simulink model "power_pmmotor"  (R2013a)
settings: Solver=ode23tb  SolverMode=SingleTasking  StartTime=0.0  StopTime=0.06  RelTol=1e-4
libraries: powerlib x5
Description:
  | Copyright 2008-2013 The MathWorks, Inc.
settings Model: ExtModeTrigMode=oneshot  ExtModeArmWhenConnect=off  ExtModeAutoUpdateStatusClock=off  Creator=MathWorks  LastModifiedBy=batserve
settings DataIOCC: ExternalInput=[]  LimitDataPoints=off  SignalLoggingSaveFormat=ModelDataLogs  SaveOutput=off  SaveTime=off  SignalLoggingName=sigsOut
settings OptimizationCC: BlockReduction=off  BooleanDataType=off  ExpressionDepthLimit=2147483647  InitFltsAndDblsToZero=on  EfficientMapNaN2IntZero=off
settings DebuggingCC: CheckExecutionContextPreStartOutputMsg=on  CheckExecutionContextRuntimeOutputMsg=on  SignalResolutionControl=TryResolveAllWithWarning  SolverPrmCheckMsg=none  MultiTaskDSMMsg=warning  MultiTaskCondExecSysMsg=none  SigSpecEnsureSampleTimeMsg=none  FcnCallInpInsideContextMsg=UseLocalSettings
settings HardwareCC: TargetUnknown=on
settings RTWCC: IncludeERTFirstTime=on
settings GRTTargetCC: CombineOutputUpdateFcns=off  GRTInterface=on

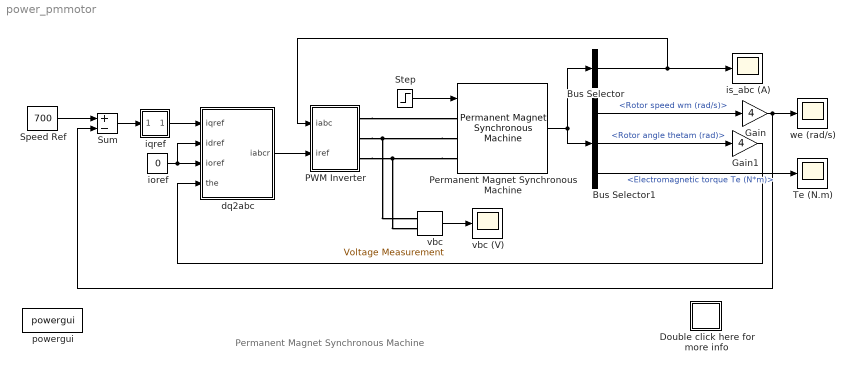
== system power_pmmotor ==
  note: Permanent Magnet Synchronous Machine
  Bus Selector : BusSelector  OutputSignals=Stator current is_a (A),Stator current is_b (A),Stator current is_c (A)  OutputAsBus=on
  Bus Selector1 : BusSelector  OutputSignals=Rotor speed wm (rad/s),Rotor angle thetam (rad),Electromagnetic torque Te (N*m)
  Double click here for more info : Subsystem
      settings: OpenFcn=showdemo(bdroot(gcb))
      mask Display: disp('?')
  Gain : Gain  Gain=4  SaturateOnIntegerOverflow=on  OutDataTypeStr=Inherit: Same as input  ParamDataTypeStr=Inherit: Same as input
  Gain1 : Gain  Gain=4  SaturateOnIntegerOverflow=on  OutDataTypeStr=Inherit: Same as input  ParamDataTypeStr=Inherit: Same as input
  PWM Inverter : Subsystem
  Permanent Magnet Synchronous Machine : powerlib/Machines/Permanent Magnet Synchronous Machine  NbPhases=3  FluxDistribution=Sinusoidal  RotorType=Round  MechanicalLoad=Torque Tm  PresetModel=No  ShowDetailedParameters=on  Resistance=2.875  Inductance=8.5e-3  dqInductances=[8.5e-3,8.5e-3]  La=0.00153  MachineConstant=Flux linkage established by magnets (V.s)  Flux=0.175  VoltageCst=126.966  TorqueCst=1.05  Flat=120  Mechanical=[ 0.8e-3, 0 4]  PolePairs=4  InitialConditions=[0,0, 0,0]  InitialConditions5ph=[0 0 0 0 0 0]  TsPowergui=0  TsBlock=-1  RefAngle=90 degrees behind phase A axis (modified Park)
  Speed Ref : Constant  Value=700
  Step : Step  Time=0.04  Before=3  SampleTime=0
  Sum : Sum  Inputs=+-  SaturateOnIntegerOverflow=on  InputSameDT=on  OutDataTypeStr=Inherit: Same as first input
  Te (N.m) : Scope
      settings: TimeRange=0.06  YMin=-20  YMax=35  DataFormat=Structure
  dq2abc : Subsystem
  ioref : Constant  Value=0
  iqref : Subsystem  mask(PI Controller){I=3, P=40, sat=[-30, 30]}
      mask prompts: I "Integral"; P "Proportional:"; sat "Minimum and maximum outputs:"
      mask init:
      | min=sat(1);max=sat(2);
      mask Display: disp('PI')
  is_abc (A) : Scope
      settings: TimeRange=0.06  YMin=-30  YMax=35  DataFormat=Structure
  powergui : powerlib/powergui  SimulationMode=Continuous  SolverType=Tustin  SampleTime=0  frequency=60  SPID=off  DisableSnubberDevices=off  DisableRonSwitches=off  DisableVfSwitches=off  SwTol=0  Interpol=off  DisplayEquations=off  frequencyindice=0  Pbase=100e6  ErrMax=1e-4  Iterations=50  UnitsV=kV  UnitsW=MW  FunctionMessages=off  echomessages=off  HookPort=off  EnableUseOfTLC=off  x0status=blocks  RestoreLinks=warning  ResistiveCurrentMeasurement=off  Frange=[0:2:500]  Ylog=off  Xlog=on  ShowGrid=off  save=off  variable=ZData  ZoomFFT=on  StartTime=0.0  cycles=1  DisplayStyle=1  fundamental=60  FreqAxis=off  MaxFrequency=1000  frequencyindicesteady=1  RmsSteady=1  display=off  Ts=0  methode=off
  vbc : powerlib/Measurements/Voltage Measurement  Tag=PoWeRsYsTeMmEaSuReMeNt  PhasorSimulation=off  OutputType=Magnitude  PSBequivalent=0
  vbc (V) : Scope
      settings: TimeRange=0.06  YMin=-500  YMax=500  DataFormat=Structure
  we (rad/s) : Scope
      settings: TimeRange=0.06  YMin=0  YMax=800  DataFormat=Structure
  wires:
  ioref/1 -> dq2abc/2(idref), dq2abc/3(ioref)
  Sum/1 -> iqref/1(In_1)
  Speed Ref/1 -> Sum/1
  iqref/1(Out_1) -> dq2abc/1(iqref)
  dq2abc/1(iabcr) -> PWM Inverter/2(iref)
  Bus Selector1/3 -> Te (N.m)/1  "<Electromagnetic torque Te (N*m)>"
  Gain/1 -> we (rad/s)/1, Sum/2
  Gain1/1 -> dq2abc/4(the)
  Step/1 -> Permanent Magnet Synchronous Machine/1
  Permanent Magnet Synchronous Machine/1 -> Bus Selector/1, Bus Selector1/1
  vbc/1 -> vbc (V)/1
  Bus Selector/1 -> PWM Inverter/1(iabc), is_abc (A)/1
  Bus Selector1/1 -> Gain/1  "<Rotor speed wm (rad/s)>"
  Bus Selector1/2 -> Gain1/1  "<Rotor angle thetam (rad)>"
  connections:
  PWM Inverter/RConn1 -- Permanent Magnet Synchronous Machine/LConn1
  Permanent Magnet Synchronous Machine/LConn2 -- PWM Inverter/RConn2 -- vbc/LConn1
  Permanent Magnet Synchronous Machine/LConn3 -- PWM Inverter/RConn3 -- vbc/LConn2

== system power_pmmotor/Double click here for more info ==

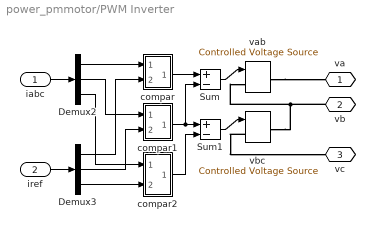
== system power_pmmotor/PWM Inverter ==
  iabc : Inport
  iref : Inport  Port=2
  Demux2 : Demux  Outputs=3
  Demux3 : Demux  Outputs=3
  Sum : Sum  Inputs=+-  SaturateOnIntegerOverflow=on  InputSameDT=on  OutDataTypeStr=Inherit: Same as first input
  Sum1 : Sum  Inputs=+-  SaturateOnIntegerOverflow=on  InputSameDT=on  OutDataTypeStr=Inherit: Same as first input
  compar : Subsystem
  compar1 : Subsystem
  compar2 : Subsystem
  vab : powerlib/Electrical Sources/Controlled Voltage Source  Description=source block  Initialize=on  Source_Type=AC  Amplitude=0  Phase=0  Frequency=0  Measurements=None
      settings: AttributesFormatString=\n
  vbc : powerlib/Electrical Sources/Controlled Voltage Source  Description=source block  Initialize=on  Source_Type=AC  Amplitude=0  Phase=0  Frequency=0  Measurements=None
      settings: AttributesFormatString=\n
  va : PMIOPort  Port=1  Side=Right
  vb : PMIOPort  Port=2  Side=Right
  vc : PMIOPort  Port=3  Side=Right
  wires:
  Demux2/1 -> compar/1(ia)
  Demux2/2 -> compar1/1(ib)
  Demux2/3 -> compar2/1(ic)
  Demux3/3 -> compar2/2(icr)
  Demux3/2 -> compar1/2(ibr)
  Demux3/1 -> compar/2(iar)
  compar/1(va) -> Sum/1
  compar1/1(vb) -> Sum/2, Sum1/1
  compar2/1(vc) -> Sum1/2
  iabc/1 -> Demux2/1
  iref/1 -> Demux3/1
  Sum/1 -> vab/1
  Sum1/1 -> vbc/1
  connections:
  vab/RConn1 -- va/RConn1
  vb/RConn1 -- vab/LConn1 -- vbc/RConn1
  vbc/LConn1 -- vc/RConn1

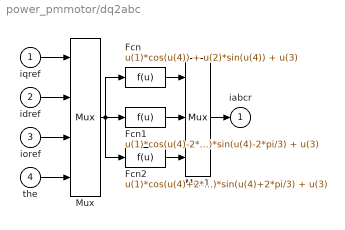
== system power_pmmotor/dq2abc ==
  iqref : Inport
  idref : Inport  Port=2
  ioref : Inport  Port=3
  the : Inport  Port=4
  Fcn : Fcn  Expr=u(1)*cos(u(4)) + u(2)*sin(u(4)) + u(3)
  Fcn1 : Fcn  Expr=u(1)*cos(u(4)-2*pi/3) + u(2)*sin(u(4)-2*pi/3) + u(3)
  Fcn2 : Fcn  Expr=u(1)*cos(u(4)+2*pi/3) + u(2)*sin(u(4)+2*pi/3) + u(3)
  Mux : Mux
  Mux1 : Mux  Inputs=3
  iabcr : Outport  InitialOutput=0
  wires:
  the/1 -> Mux/4
  ioref/1 -> Mux/3
  idref/1 -> Mux/2
  iqref/1 -> Mux/1
  Mux/1 -> Fcn1/1, Fcn2/1, Fcn/1
  Fcn1/1 -> Mux1/2
  Fcn/1 -> Mux1/1
  Fcn2/1 -> Mux1/3
  Mux1/1 -> iabcr/1

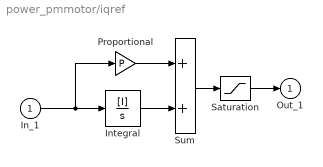
== system power_pmmotor/iqref ==
  In_1 : Inport
  Integral : TransferFcn  Numerator=[I]  Denominator=[1 0]
  Proportional : Gain  Gain=P  SaturateOnIntegerOverflow=on  OutDataTypeStr=Inherit: Same as input  ParamDataTypeStr=Inherit: Same as input
  Saturation : Saturate  UpperLimit=max  LowerLimit=min
  Sum : Sum  SaturateOnIntegerOverflow=on  InputSameDT=on  OutDataTypeStr=Inherit: Same as first input
  Out_1 : Outport  InitialOutput=0
  wires:
  Integral/1 -> Sum/2
  In_1/1 -> Integral/1, Proportional/1
  Proportional/1 -> Sum/1
  Sum/1 -> Saturation/1
  Saturation/1 -> Out_1/1

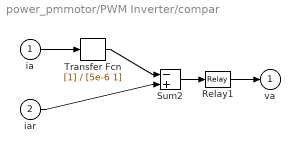
== system power_pmmotor/PWM Inverter/compar ==
  ia : Inport
  iar : Inport  Port=2
  Relay1 : Relay  OnSwitchValue=0.05  OffSwitchValue=-0.05  OnOutputValue=155  OffOutputValue=-155
  Sum2 : Sum  Inputs=-+  SaturateOnIntegerOverflow=on  InputSameDT=on  OutDataTypeStr=Inherit: Same as first input
  Transfer Fcn : TransferFcn  Denominator=[5e-6 1]
  va : Outport  InitialOutput=0
  wires:
  iar/1 -> Sum2/2
  Sum2/1 -> Relay1/1
  Relay1/1 -> va/1
  ia/1 -> Transfer Fcn/1
  Transfer Fcn/1 -> Sum2/1

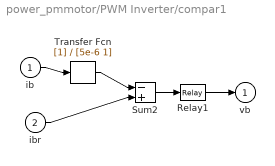
== system power_pmmotor/PWM Inverter/compar1 ==
  ib : Inport
  ibr : Inport  Port=2
  Relay1 : Relay  OnSwitchValue=0.05  OffSwitchValue=-0.05  OnOutputValue=155  OffOutputValue=-155
  Sum2 : Sum  Inputs=-+  SaturateOnIntegerOverflow=on  InputSameDT=on  OutDataTypeStr=Inherit: Same as first input
  Transfer Fcn : TransferFcn  Denominator=[5e-6 1]
  vb : Outport  InitialOutput=0
  wires:
  ibr/1 -> Sum2/2
  Sum2/1 -> Relay1/1
  Relay1/1 -> vb/1
  ib/1 -> Transfer Fcn/1
  Transfer Fcn/1 -> Sum2/1

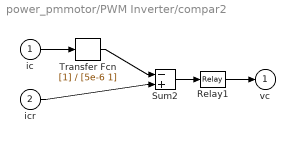
== system power_pmmotor/PWM Inverter/compar2 ==
  ic : Inport
  icr : Inport  Port=2
  Relay1 : Relay  OnSwitchValue=0.05  OffSwitchValue=-0.05  OnOutputValue=155  OffOutputValue=-155
  Sum2 : Sum  Inputs=-+  SaturateOnIntegerOverflow=on  InputSameDT=on  OutDataTypeStr=Inherit: Same as first input
  Transfer Fcn : TransferFcn  Denominator=[5e-6 1]
  vc : Outport  InitialOutput=0
  wires:
  icr/1 -> Sum2/2
  Sum2/1 -> Relay1/1
  Relay1/1 -> vc/1
  ic/1 -> Transfer Fcn/1
  Transfer Fcn/1 -> Sum2/1
